simulink model "test_lan"  (Simulink 7.6)
settings: Solver=FixedStepDiscrete  StartTime=0.0  StopTime=3000  FixedStep=1  RelTol=1e-3
libraries: simulink x3
settings Model: Creator=jordan  LastModifiedBy=jordan
settings DataIOCC: LimitDataPoints=off  SaveOutput=off  SignalLogging=off  DSMLogging=off  SaveTime=off
settings OptimizationCC: BlockReduction=off  ConditionallyExecuteInputs=off  InlineParams=on

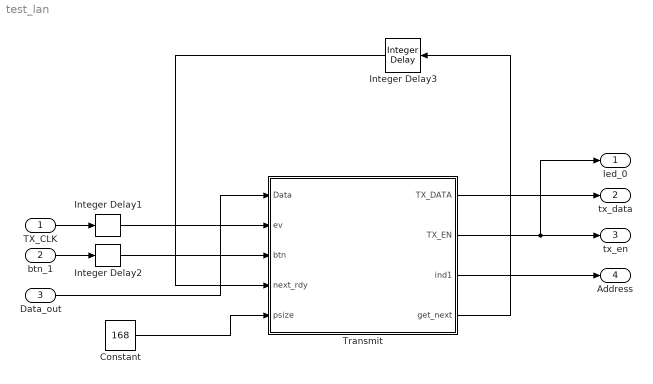
== system test_lan ==
  TX_CLK : Inport  OutDataTypeStr=boolean
  btn_1 : Inport  Port=2  OutDataTypeStr=boolean
  Data_out : Inport  Port=3  OutDataTypeStr=uint8
  Constant : Constant  Value=168  OutDataTypeStr=Inherit: Inherit via back propagation
  Integer Delay1 : simulink/Discrete/Integer Delay  NumDelays=1  vinit=0.0  samptime=-1
  Integer Delay2 : simulink/Discrete/Integer Delay  NumDelays=1  vinit=0.0  samptime=-1
  Integer Delay3 : simulink/Discrete/Integer Delay  NumDelays=1  vinit=0.0  samptime=-1
  Transmit : Stateflow chart  TreatAsAtomicUnit=on
  led_0 : Outport
  tx_data : Outport  Port=2
  tx_en : Outport  Port=3
  Address : Outport  Port=4
  wires:
  Transmit/1(TX_DATA) -> tx_data/1
  Transmit/2(TX_EN) -> led_0/1, tx_en/1
  Transmit/3(ind1) -> Address/1
  Transmit/4(get_next) -> Integer Delay3/1
  Integer Delay3/1 -> Transmit/4(next_rdy)
  TX_CLK/1 -> Integer Delay1/1
  btn_1/1 -> Integer Delay2/1
  Integer Delay1/1 -> Transmit/2(ev)
  Integer Delay2/1 -> Transmit/3(btn)
  Data_out/1 -> Transmit/1(Data)
  Constant/1 -> Transmit/5(psize)

== stateflow chart Transmit ==
  settings: executeAtInitialization=1
  state Wait10
  state Start_tx
  state Wait14
  state Wait_for_ev
  state Wait12
  state Get_Data
  state Data_Ready
  state Wait13
  state move8crc [function]
    (default) -> (junction 17) : {ind2=0;}
    (junction 17) -> (junction 19) : {buf_bit=CRC>>31;
        | CRC=CRC<<1;
        | buf32=buf_tx; buf32=buf32>>ind2;
        | buf32=buf32&1;
        | CRC=CRC|buf32;
        | ind2++;}
    (junction 19) -> (junction 20) [order 1] : [buf_bit]{CRC=CRC^gen_poly;}
    (junction 19) -> (junction 20) [order 2]
    (junction 25) -> (junction 24) [order 2]
    (junction 25) -> (junction 24) [order 1] : [buf_bit]{CRC=CRC^gen_poly;}
    (junction 20) -> (junction 25) : {buf_bit=CRC>>31;
        | CRC=CRC<<1;
        | buf32=buf_tx; buf32=buf32>>ind2;
        | buf32=buf32&1;
        | CRC=CRC|buf32;
        | ind2++;}
    (junction 18) -> (junction 26) [order 2]
    (junction 18) -> (junction 26) [order 1] : [buf_bit]{CRC=CRC^gen_poly;}
    (junction 24) -> (junction 18) : {buf_bit=CRC>>31;
        | CRC=CRC<<1;
        | buf32=buf_tx; buf32=buf32>>ind2;
        | buf32=buf32&1;
        | CRC=CRC|buf32;
        | ind2++;}
    (junction 28) -> (junction 27) [order 2]
    (junction 28) -> (junction 27) [order 1] : [buf_bit]{CRC=CRC^gen_poly;}
    (junction 26) -> (junction 28) : {buf_bit=CRC>>31;
        | CRC=CRC<<1;
        | buf32=buf_tx; buf32=buf32>>ind2;
        | buf32=buf32&1;
        | CRC=CRC|buf32;
        | ind2++;}
    (junction 30) -> (junction 29) [order 2]
    (junction 30) -> (junction 29) [order 1] : [buf_bit]{CRC=CRC^gen_poly;}
    (junction 27) -> (junction 30) : {buf_bit=CRC>>31;
        | CRC=CRC<<1;
        | buf32=buf_tx; buf32=buf32>>ind2;
        | buf32=buf32&1;
        | CRC=CRC|buf32;
        | ind2++;}
    (junction 32) -> (junction 31) [order 2]
    (junction 32) -> (junction 31) [order 1] : [buf_bit]{CRC=CRC^gen_poly;}
    (junction 29) -> (junction 32) : {buf_bit=CRC>>31;
        | CRC=CRC<<1;
        | buf32=buf_tx; buf32=buf32>>ind2;
        | buf32=buf32&1;
        | CRC=CRC|buf32;
        | ind2++;}
    (junction 34) -> (junction 33) [order 2]
    (junction 34) -> (junction 33) [order 1] : [buf_bit]{CRC=CRC^gen_poly;}
    (junction 31) -> (junction 34) : {buf_bit=CRC>>31;
        | CRC=CRC<<1;
        | buf32=buf_tx; buf32=buf32>>ind2;
        | buf32=buf32&1;
        | CRC=CRC|buf32;
        | ind2++;}
    (junction 36) -> (junction 35) [order 2]
    (junction 36) -> (junction 35) [order 1] : [buf_bit]{CRC=CRC^gen_poly;}
    (junction 33) -> (junction 36) : {buf_bit=CRC>>31;
        | CRC=CRC<<1;
        | buf32=buf_tx; buf32=buf32>>ind2;
        | buf32=buf32&1;
        | CRC=CRC|buf32;
        | ind2++;}
  state CRC_end
  state Wait_for_ev1
  note: CRC initial value is first 4 bytes of destination
      | address, complemented and bit-reversed.
  (default) -> Start_tx
  Data_Ready -> (junction 16) : [ev==0]
  (junction 15) -> Wait_for_ev : {TX_DATA[0]=buf_tx&1;
      | TX_DATA[1]=buf_tx&2;
      | TX_DATA[2]=buf_tx&4;
      | TX_DATA[3]=buf_tx&8;}
  Wait13 -> Wait14 : [ev==0]{
      | TX_DATA[0]=buf_tx&16;
      | TX_DATA[1]=buf_tx&32;
      | TX_DATA[2]=buf_tx&64;
      | TX_DATA[3]=buf_tx&128;}
  (junction 21) -> Get_Data [order 1] : /*68*/[ind1<psize]{get_next=1;}
  (junction 22) -> Wait10 [order 2] : {TX_EN=0;}
  Wait10 -> Start_tx : [btn==0]
  Start_tx -> Wait12 : [btn==1]{
      | TX_EN=0;
      | get_next=0;
      | CRC=4095471226;}
  Wait12 -> Get_Data : {get_next=1;}
  Get_Data -> (junction 23) : [next_rdy==1]{
      | buf_tx=Data;
      | get_next=0;}
  Wait_for_ev -> Wait13 : [ev==1]
  (junction 16) -> (junction 15) [order 1] : [TX_EN==0]{ind1=0;TX_EN=1;}
  (junction 16) -> (junction 15) [order 2]
  (junction 23) -> Data_Ready [order 1] : /*11*/[ind1>11]{move8crc();}
  (junction 23) -> Data_Ready [order 2]
  Wait14 -> (junction 21) : [ev==1]{ind1++;}
  (junction 21) -> CRC_end [order 2] : {buf_tx=0;
      | move8crc();
      | move8crc();
      | move8crc();
      | move8crc();
      | ind1=0;
      | CRC=~CRC}
  CRC_end -> (junction 22) : [ev==0]
  Wait_for_ev1 -> CRC_end : [ev==1]{ind1++;}
  (junction 22) -> Wait_for_ev1 [order 1] : [ind1<8]{
      | TX_DATA[0]=CRC>>31;
      | TX_DATA[1]=(CRC>>30)&1;
      | TX_DATA[2]=(CRC>>29)&1;
      | TX_DATA[3]=(CRC>>28)&1;
      | CRC=CRC<<4;}
  data: Data input uint8 =0; TX_DATA output boolean size=4 =0; TX_EN output boolean =1; ind1 output fixdt(0,11,0); ev input boolean; btn input boolean; CRC local uint32; get_next output boolean; next_rdy input boolean; buf_tx local uint8; ind2 local uint8; buf_bit local boolean; gen_poly constant uint32 =79764919; buf32 local uint32; psize input fixdt(0,11,0)
  data Data settings: description=8 bit data, little endian
